simulink model "tablica"  (R2023b)
settings: Solver=FixedStepAuto  StartTime=0.0  StopTime=10.0  FixedStep=0.001  RelTol=1e-3
settings Model: Creator=majaw  LastModifiedBy=majaw

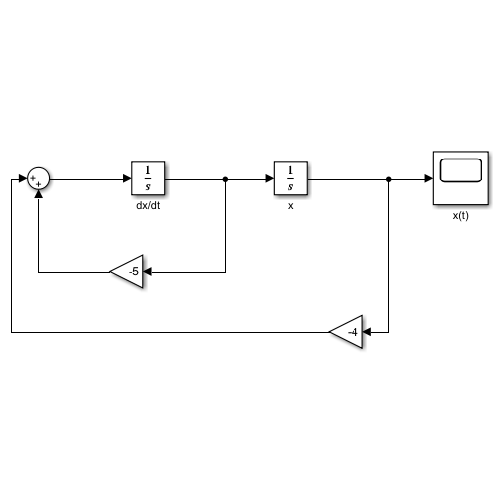
[thumbnail: Simulink's stored preview of the top-level diagram]
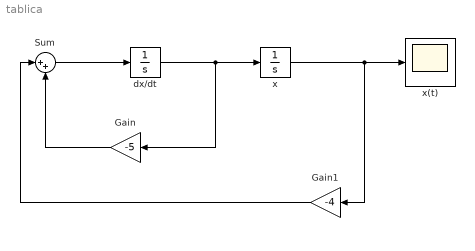
== system tablica ==
  Gain : Gain  Gain=-5
  Gain1 : Gain  Gain=-4
  Sum : Sum  Inputs=|++
  dx/dt : Integrator  InitialCondition=1
  x : Integrator
  x(t) : Scope
  wires:
  Sum/1 -> dx/dt/1
  dx/dt/1 -> Gain/1, x/1
  x/1 -> Gain1/1, x(t)/1
  Gain/1 -> Sum/2
  Gain1/1 -> Sum/1
